simulink model "some_simulation"  (R2016a)
settings: Solver=VariableStepAuto  StartTime=0.0  StopTime=100  RelTol=1e-3
libraries: simulink x2
settings Model: Creator=古乔  LastModifiedBy=古乔

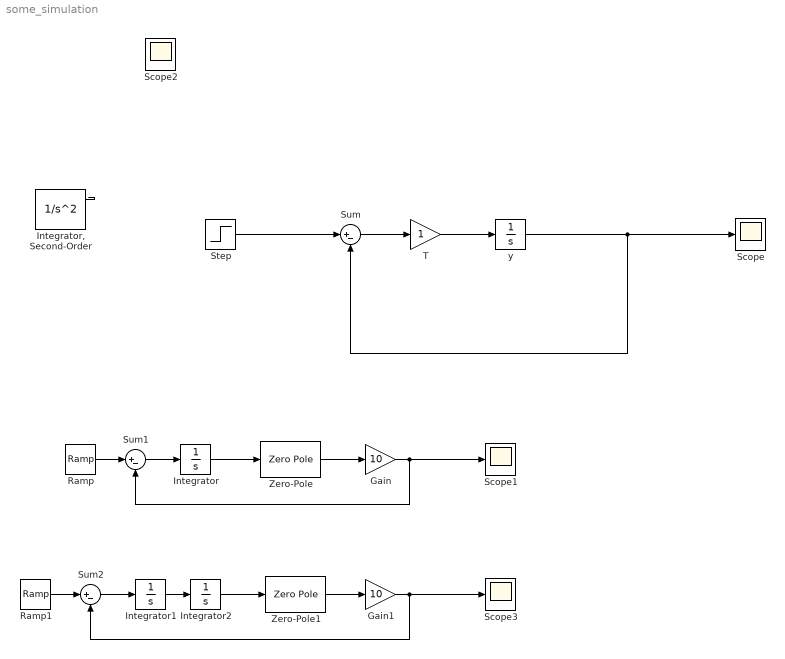
== system some_simulation ==
  Gain : Gain  Gain=10
  Gain1 : Gain  Gain=10
  Integrator : Integrator
  "Integrator, Second-Order" : SecondOrderIntegrator
  Integrator1 : Integrator
  Integrator2 : Integrator
  Ramp : simulink/Sources/Ramp  slope=1  start=0  X0=0
  Ramp1 : simulink/Sources/Ramp  slope=1  start=0  X0=0
  Scope{,1..3} (4 alike) : Scope
  Step : Step  SampleTime=0
  Sum : Sum  Inputs=|+-
  Sum1 : Sum  Inputs=|+-
  Sum2 : Sum  Inputs=|+-
  T : Gain
  Zero-Pole : ZeroPole  Zeros=[]  Poles=[-10 -1]
  Zero-Pole1 : ZeroPole  Zeros=[]  Poles=[-10 -1]
  y : Integrator
  wires:
  Step/1 -> Sum/1
  y/1 -> Scope/1, Sum/2
  T/1 -> y/1
  Sum/1 -> T/1
  Ramp/1 -> Sum1/1
  Integrator/1 -> Zero-Pole/1
  Zero-Pole/1 -> Gain/1
  Gain/1 -> Sum1/2, Scope1/1
  Sum1/1 -> Integrator/1
  Ramp1/1 -> Sum2/1
  "Integrator, Second-Order"/1 -> ?
  Zero-Pole1/1 -> Gain1/1
  Gain1/1 -> Sum2/2, Scope3/1
  Sum2/1 -> Integrator1/1
  Integrator1/1 -> Integrator2/1
  Integrator2/1 -> Zero-Pole1/1
